simulink model "bh_COMPONENT_U_rectangular_pulse"  (R2026b)
settings: Solver=VariableStepAuto
settings Model: Creator=bhorton  LastModifiedBy=bhorton

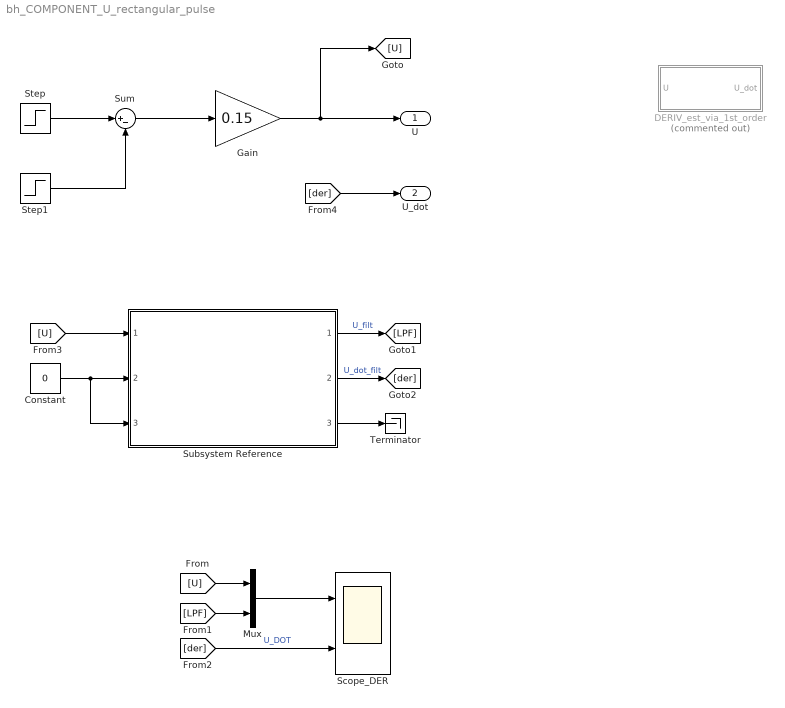
== system bh_COMPONENT_U_rectangular_pulse ==
  Constant : Constant  Value=0
  DERIV_est_via_1st_order : Subsystem  Commented=on
  Gain : Gain  Gain=0.15
  Mux : Mux  Inputs=2
  Scope_DER : Scope  NumInputPorts=2
      settings: ActiveDisplayYMinimum=-0.0099363483435303546  ActiveDisplayYMaximum=0.15737486679996648  DataLoggingVariableName=ScopeData2
  Step : Step  Time=3  SampleTime=0
      settings: AttributesFormatString=Step TIME = %<Time> (secs)
  Step1 : Step  Time=8  SampleTime=0
      settings: AttributesFormatString=Step TIME = %<Time> (secs)
  Subsystem Reference : Subsystem  ReferencedSubsystem=bh_COMPONENT_deriv_est  wn=2*pi*150  p=1
  Sum : Sum  Inputs=|+-
  Terminator : Terminator
  U : Outport
  U_dot : Outport  Port=2
  wires:
  Step/1 -> Sum/1
  Step1/1 -> Sum/2
  Sum/1 -> Gain/1
  Gain/1 -> U/1, [U]
  [U] -> Mux/1
  [LPF] -> Mux/2
  [der] -> Scope_DER/2  "U_DOT"
  Mux/1 -> Scope_DER/1
  [U] -> Subsystem Reference/1
  Constant/1 -> Subsystem Reference/2, Subsystem Reference/3
  Subsystem Reference/1 -> [LPF]  "U_filt"
  Subsystem Reference/2 -> [der]  "U_dot_filt"
  Subsystem Reference/3 -> Terminator/1
  [der] -> U_dot/1

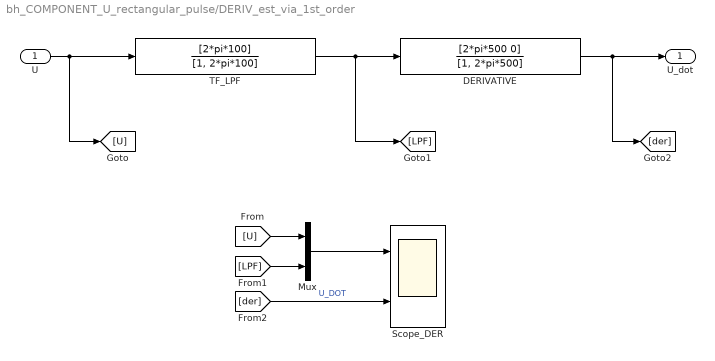
== system bh_COMPONENT_U_rectangular_pulse/DERIV_est_via_1st_order ==
  U : Inport
  DERIVATIVE : TransferFcn  Numerator=[2*pi*500 0]  Denominator=[1, 2*pi*500]
  Mux : Mux  Inputs=2
  Scope_DER : Scope  NumInputPorts=2
      settings: ActiveDisplayYMinimum=-0.01875  ActiveDisplayYMaximum=0.16875
  TF_LPF : TransferFcn  Numerator=[2*pi*100]  Denominator=[1, 2*pi*100]
  U_dot : Outport
  wires:
  TF_LPF/1 -> DERIVATIVE/1, [LPF]
  DERIVATIVE/1 -> U_dot/1, [der]
  Mux/1 -> Scope_DER/1
  [LPF] -> Mux/2
  U/1 -> TF_LPF/1, [U]
  [U] -> Mux/1
  [der] -> Scope_DER/2  "U_DOT"
